simulink model "q4_2"  (R2019a)
settings: Solver=FixedStepAuto  StartTime=0.0  StopTime=0.01  FixedStep=1e-8  RelTol=1e-3
libraries: dsparch4 x2
settings Model: Creator=marco  LastModifiedBy=marco

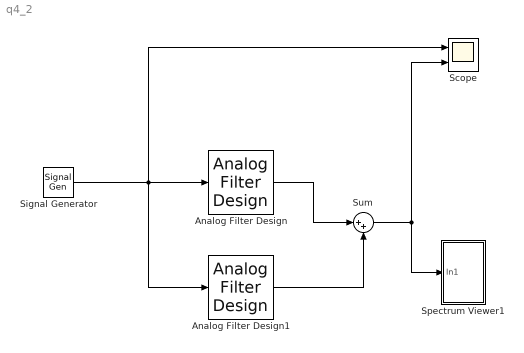
== system q4_2 ==
  Analog Filter Design : dsparch4/Analog Filter Design  method=Butterworth  filttype=Highpass  N=3  Wlo=2*pi*2e6  Whi=80  Rp=2  Rs=40
  Analog Filter Design1 : dsparch4/Analog Filter Design  method=Butterworth  filttype=Lowpass  N=3  Wlo=2*pi*1e6  Whi=80  Rp=2  Rs=40
  Scope : Scope  NumInputPorts=2
  Signal Generator : SignalGenerator  WaveForm=square  Frequency=1e5
  Spectrum Viewer1 : Subsystem
  Sum : Sum  Inputs=|++
  wires:
  Signal Generator/1 -> Analog Filter Design1/1, Scope/1, Analog Filter Design/1
  Analog Filter Design1/1 -> Sum/2
  Analog Filter Design/1 -> Sum/1
  Sum/1 -> Spectrum Viewer1/1(In1), Scope/2

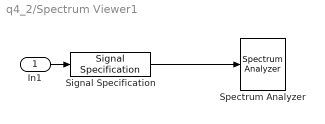
== system q4_2/Spectrum Viewer1 ==
  In1 : Inport
  Signal Specification : SignalSpecification  SampleTime=1e-7
  Spectrum Analyzer : SpectrumAnalyzer
  wires:
  In1/1 -> Signal Specification/1
  Signal Specification/1 -> Spectrum Analyzer/1
